simulink model "Pedal_Position_Sensor"  (R2021a)
settings: Solver=FixedStepAuto  StartTime=0.0  StopTime=10.0  RelTol=1e-3
libraries: simulink x3, pil_lib x2
settings Model: Creator=LenovoID3  LastModifiedBy=LenovoID3
settings OptimizationCC: DefaultParameterBehavior=Inlined  EnhancedBackFolding=on  PassReuseOutputArgsAs=Individual arguments  ZeroExternalMemoryAtStartup=off  ZeroInternalMemoryAtStartup=off  OptimizeBlockOrder=speed  DifferentSizesBufferReuse=on  OptimizationCustomize=off  EfficientTunableParamExpr=on
settings DebuggingCC: ParameterTunabilityLossMsg=error
settings SFSimCC: MATLABDynamicMemAlloc=off
settings RTWCC: SystemTargetFile=ert.tlc  TemplateMakefile=ert_default_tmf  CreateSILPILBlock=SIL
settings CodeAppCC: ForceParamTrailComments=on  IgnoreCustomStorageClasses=off  OperatorAnnotations=on  SimulinkDataObjDesc=on  SFDataObjDesc=on  InsertBlockDesc=on
settings ERTTargetCC: TargetLangStandard=C99 (ISO)  GenerateSampleERTMain=on  SupportContinuousTime=on  InlinedParameterPlacement=NonHierarchical  ERTCustomFileTemplate=example_file_process.tlc

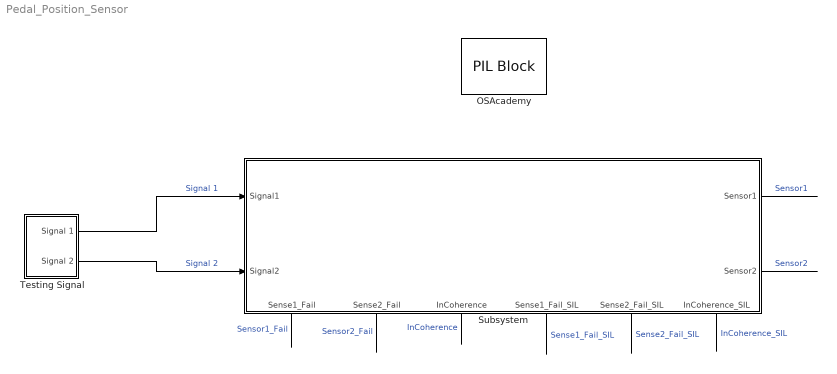
== system Pedal_Position_Sensor ==
  OSAcademy : pil_lib/PIL Block  SimulationMode=SIL  IsTopModelPIL=off  CodeDir=C:\Users\LenovoID3\Downloads\New folder\OSAcademy_ert_rtw  AnchorDir=C:\Users\LenovoID3\Downloads\New folder  ConfigName=Software-in-the-Loop (SIL)  XrelIsTopModelCode=on  XrelIsReusable=off  XrelDWorkNames={}  XrelDWorkTypes={}  XrelModelArgVals={}  XrelOrderedParamNames={}
      settings: SourceProductBaseCode=RT
  Subsystem : Subsystem
      settings: PortSchema="{\"entries\":[{\"content\":{\"sides\":[{\"content\":{\"connectorIds\":[\"In1\",\"In2\"]},\"type\":\"ConnectorPlacement.EquallySpacedRectSide\",\"uuid\":\"b8229edd-deda-40cf-ad5a-24b3db798bf7\"},{\"content\":{\"connectorIds\":[\"Out1\",\"Out2\"],\"side\":\"RIGHT\"},\"type\":\"ConnectorPlacement.EquallySpacedRectSide\",\"uuid\":\"8a2a6cfd-0422-46e1-aba6-13dd86feb93d\"},{\"content\":{\"connectorIds\":[],\"side\":\"TOP\"},\"type\":\"ConnectorPlacement.EquallySpacedRectSide\",\"uuid\":\"1ebd3a65-a67e-4261-83c1-f99d1798de09\"},{\"content\":{\"connectorIds\":[\"Out3\",\"Out4\",\"Out5\",\"Out6\",\"Out7\",\"Out8\"],\"side\":\"BOTTOM\"},\"type\":\"ConnectorPlacement.EquallySpacedRectSide\",\"uuid\":\"0ad3b253-8be6-4aef-90be-6048caeda625\"}]},\"type\":\"ConnectorPlacement.EquallySpacedConnector\",\"uuid\":\"11bd23d5-d2a7-463d-b28b-d598d29700f0\"}],\"packageUris\":[\"http://schema.mathworks.com/mf0/Connector/R2020b\"],\"version\":\"1.0\"}"
  Testing Signal : Subsystem
  wires:
  Subsystem/1(Sensor1) -> ?  "Sensor1"
  Subsystem/2(Sensor2) -> ?  "Sensor2"
  Subsystem/5(InCoherence) -> ?  "InCoherence"
  Subsystem/4(Sense2_Fail) -> ?  "Sensor2_Fail"
  Subsystem/3(Sense1_Fail) -> ?  "Sensor1_Fail"
  Subsystem/6(Sense1_Fail_SIL) -> ?  "Sense1_Fail_SIL"
  Subsystem/7(Sense2_Fail_SIL) -> ?  "Sense2_Fail_SIL"
  Subsystem/8(InCoherence_SIL) -> ?  "InCoherence_SIL"
  Testing Signal/1(Signal 1) -> Subsystem/1(Signal1)  "Signal 1"
  Testing Signal/2(Signal 2) -> Subsystem/2(Signal2)  "Signal 2"

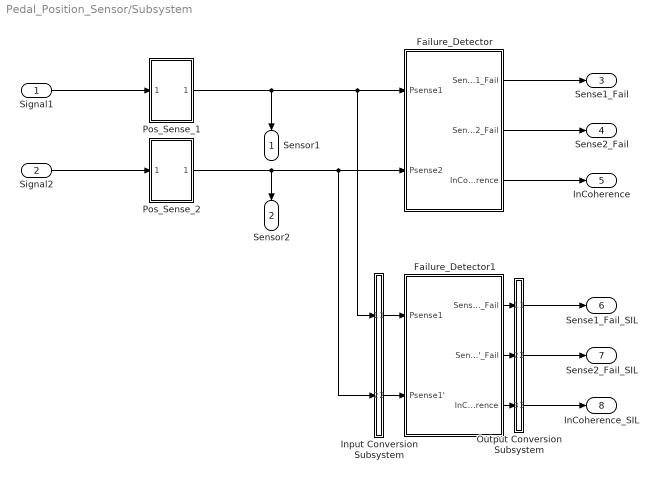
== system Pedal_Position_Sensor/Subsystem ==
  Signal1 : Inport
  Signal2 : Inport  Port=2
  Failure_Detector : Subsystem  TreatAsAtomicUnit=on
  Failure_Detector1 : Subsystem  Tag=__SL_testing_harness_stub_  DialogController=pil_create_dialog  LoadFcn=|
      | try
      |    if ~strcmp(rtw.pil.getPILVersion, '9.10 (R2021a)_15')
      |       set_param(gcb, 'DialogController', '');
      |       set_param(gcb, 'DialogControllerArgs', '');
      |    end
      | catch e
      |       set_param(gcb, 'DialogController', '');
      |       set_param(gcb, 'DialogControllerArgs', '');
      | end
      mask help: PIL:pil:XILBlockMaskDesc
      mask Display: disp('SIL');
  Input Conversion Subsystem : Subsystem  Tag=__SLT_ICS__  Description=|
      | Signal spec.
      | and routing
      settings: AttributesFormatString=%<Description>
  Output Conversion Subsystem : Subsystem  Tag=__SLT_OCS__  Description=|
      | Signal spec.
      | and routing
      settings: AttributesFormatString=%<Description>
  Pos_Sense_1 : Subsystem
  Pos_Sense_2 : Subsystem
  Sensor1 : Outport
  Sensor2 : Outport  Port=2
  Sense1_Fail : Outport  Port=3
  Sense2_Fail : Outport  Port=4
  InCoherence : Outport  Port=5
  Sense1_Fail_SIL : Outport  Port=6
  Sense2_Fail_SIL : Outport  Port=7
  InCoherence_SIL : Outport  Port=8
  wires:
  Failure_Detector/1(Sense1_Fail) -> Sense1_Fail/1
  Pos_Sense_2/1(Psense2) -> Sensor2/1, Input Conversion Subsystem/2(Inport_2), Failure_Detector/2(Psense2)
  Pos_Sense_1/1(Psense1) -> Sensor1/1, Input Conversion Subsystem/1(Inport_1), Failure_Detector/1(Psense1)
  Signal1/1 -> Pos_Sense_1/1(Input)
  Failure_Detector/3(InCoherence) -> InCoherence/1
  Failure_Detector/2(Sense2_Fail) -> Sense2_Fail/1
  Signal2/1 -> Pos_Sense_2/1(Input)
  Input Conversion Subsystem/2(Outport_2) -> Failure_Detector1/2(Psense1')
  Failure_Detector1/3(InCoherence) -> Output Conversion Subsystem/3(Inport_3)
  Output Conversion Subsystem/2(Outport_2) -> Sense2_Fail_SIL/1
  Failure_Detector1/1(Sense1_Fail) -> Output Conversion Subsystem/1(Inport_1)
  Input Conversion Subsystem/1(Outport_1) -> Failure_Detector1/1(Psense1)
  Output Conversion Subsystem/1(Outport_1) -> Sense1_Fail_SIL/1
  Output Conversion Subsystem/3(Outport_3) -> InCoherence_SIL/1
  Failure_Detector1/2(Sense1'_Fail) -> Output Conversion Subsystem/2(Inport_2)

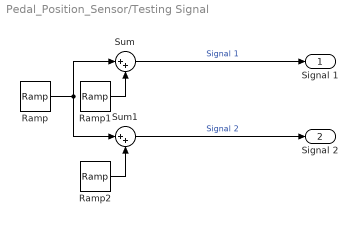
== system Pedal_Position_Sensor/Testing Signal ==
  Ramp : simulink/Sources/Ramp  slope=0.1  start=0  InitialOutput=0
  Ramp1 : simulink/Sources/Ramp  slope=0.2  start=5  InitialOutput=0
  Ramp2 : simulink/Sources/Ramp  slope=0.3  start=5  InitialOutput=0
  Sum : Sum  Inputs=|++
  Sum1 : Sum  Inputs=|++
  Signal 1 : Outport
  Signal 2 : Outport  Port=2
  wires:
  Ramp2/1 -> Sum1/2
  Ramp1/1 -> Sum/2
  Sum/1 -> Signal 1/1  "Signal 1"
  Sum1/1 -> Signal 2/1  "Signal 2"
  Ramp/1 -> Sum/1, Sum1/1

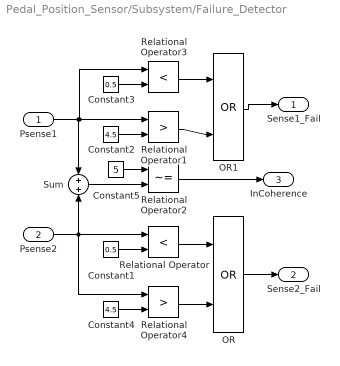
== system Pedal_Position_Sensor/Subsystem/Failure_Detector ==
  Psense1 : Inport
  Psense2 : Inport  Port=2
  Constant1 : Constant  Value=0.5
  Constant2 : Constant  Value=4.5
  Constant3 : Constant  Value=0.5
  Constant4 : Constant  Value=4.5
  Constant5 : Constant  Value=5
  OR : Logic  Operator=OR  AllPortsSameDT=off  OutDataTypeStr=boolean
  OR1 : Logic  Operator=OR  AllPortsSameDT=off  OutDataTypeStr=boolean
  Relational Operator : RelationalOperator  Operator=<  OutDataTypeStr=boolean  RndMeth=Simplest
  Relational Operator1 : RelationalOperator  Operator=>  OutDataTypeStr=boolean  RndMeth=Simplest
  Relational Operator2 : RelationalOperator  Operator=~=  OutDataTypeStr=boolean  RndMeth=Simplest
  Relational Operator3 : RelationalOperator  Operator=<  OutDataTypeStr=boolean  RndMeth=Simplest
  Relational Operator4 : RelationalOperator  Operator=>  OutDataTypeStr=boolean  RndMeth=Simplest
  Sum : Sum
  Sense1_Fail : Outport
  Sense2_Fail : Outport  Port=2
  InCoherence : Outport  Port=3
  wires:
  Constant1/1 -> Relational Operator/2
  Constant2/1 -> Relational Operator1/2
  Constant3/1 -> Relational Operator3/2
  Psense1/1 -> Relational Operator3/1, Relational Operator1/1, Sum/1
  Psense2/1 -> Relational Operator4/1, Sum/2, Relational Operator/1
  Constant4/1 -> Relational Operator4/2
  Relational Operator/1 -> OR/1
  Relational Operator4/1 -> OR/2
  Relational Operator1/1 -> OR1/2
  Relational Operator3/1 -> OR1/1
  OR1/1 -> Sense1_Fail/1
  OR/1 -> Sense2_Fail/1
  Relational Operator2/1 -> InCoherence/1
  Sum/1 -> Relational Operator2/2
  Constant5/1 -> Relational Operator2/1

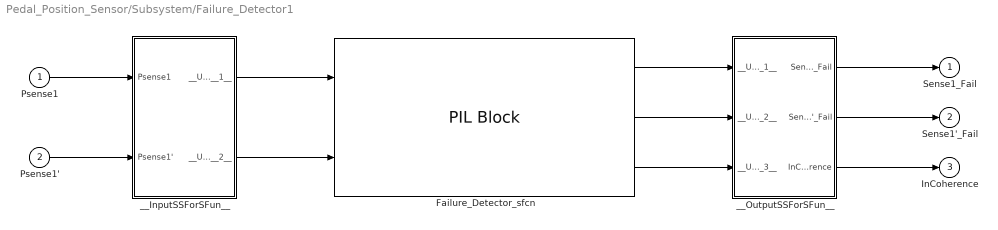
== system Pedal_Position_Sensor/Subsystem/Failure_Detector1 ==
  Psense1 : Inport
  Psense1' : Inport  Port=2
  Failure_Detector_sfcn : pil_lib/PIL Block  SimulationMode=SIL  IsTopModelPIL=off  CodeDir=C:\Users\LenovoID3\Downloads\New folder\Failure_Detector_ert_rtw  AnchorDir=C:\Users\LenovoID3\Downloads\New folder  ConfigName=Software-in-the-Loop (SIL)  XrelIsTopModelCode=on  XrelIsReusable=off  XrelDWorkNames={}  XrelDWorkTypes={}  XrelModelArgVals={}  XrelOrderedParamNames={}
      settings: SourceProductBaseCode=RT
  __InputSSForSFun__ : Subsystem
  __OutputSSForSFun__ : Subsystem
  Sense1_Fail : Outport
  Sense1'_Fail : Outport  Port=2
  InCoherence : Outport  Port=3
  wires:
  __OutputSSForSFun__/3(InCoherence) -> InCoherence/1
  __OutputSSForSFun__/2(Sense1'_Fail) -> Sense1'_Fail/1
  __OutputSSForSFun__/1(Sense1_Fail) -> Sense1_Fail/1
  Failure_Detector_sfcn/3 -> __OutputSSForSFun__/3(__UniqueInportName__3__)
  Failure_Detector_sfcn/2 -> __OutputSSForSFun__/2(__UniqueInportName__2__)
  Failure_Detector_sfcn/1 -> __OutputSSForSFun__/1(__UniqueInportName__1__)
  __InputSSForSFun__/2(__UniqueOutportName__2__) -> Failure_Detector_sfcn/2
  __InputSSForSFun__/1(__UniqueOutportName__1__) -> Failure_Detector_sfcn/1
  Psense1'/1 -> __InputSSForSFun__/2(Psense1')
  Psense1/1 -> __InputSSForSFun__/1(Psense1)

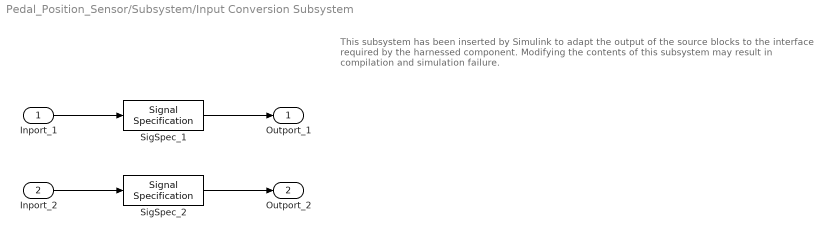
== system Pedal_Position_Sensor/Subsystem/Input Conversion Subsystem ==
  note: This subsystem has been inserted by Simulink to adapt the output of the source blocks to the interface required by the harnessed component.
      |  Modifying the contents of this subsystem may result in compilation and simulation failure.
  Inport_1 : Inport
  Inport_2 : Inport  Port=2
  SigSpec_1 : SignalSpecification  OutDataTypeStr=double  Dimensions=[1]  SampleTime=[0, 0]
  SigSpec_2 : SignalSpecification  OutDataTypeStr=double  Dimensions=[1]  SampleTime=[0, 0]
  Outport_1 : Outport
  Outport_2 : Outport  Port=2
  wires:
  SigSpec_1/1 -> Outport_1/1
  Inport_1/1 -> SigSpec_1/1
  SigSpec_2/1 -> Outport_2/1
  Inport_2/1 -> SigSpec_2/1

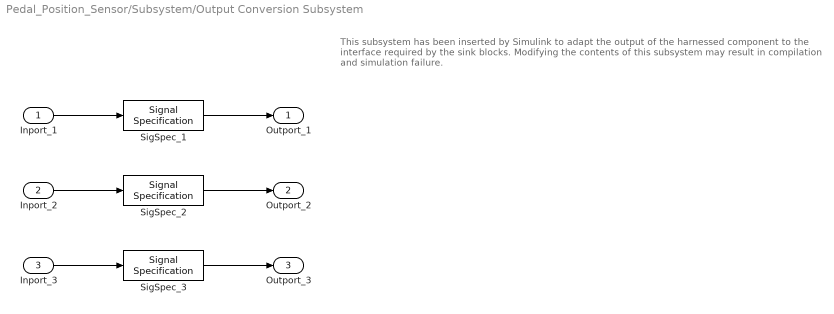
== system Pedal_Position_Sensor/Subsystem/Output Conversion Subsystem ==
  note: This subsystem has been inserted by Simulink to adapt the output of the harnessed component to the interface required by the sink blocks.
      |  Modifying the contents of this subsystem may result in compilation and simulation failure.
  Inport_1 : Inport
  Inport_2 : Inport  Port=2
  Inport_3 : Inport  Port=3
  SigSpec_1 : SignalSpecification  OutDataTypeStr=boolean  Dimensions=[1]
  SigSpec_2 : SignalSpecification  OutDataTypeStr=boolean  Dimensions=[1]
  SigSpec_3 : SignalSpecification  OutDataTypeStr=boolean  Dimensions=[1]
  Outport_1 : Outport
  Outport_2 : Outport  Port=2
  Outport_3 : Outport  Port=3
  wires:
  Inport_1/1 -> SigSpec_1/1
  SigSpec_1/1 -> Outport_1/1
  Inport_2/1 -> SigSpec_2/1
  SigSpec_2/1 -> Outport_2/1
  Inport_3/1 -> SigSpec_3/1
  SigSpec_3/1 -> Outport_3/1

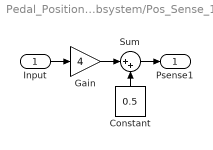
== system Pedal_Position_Sensor/Subsystem/Pos_Sense_1 ==
  Input : Inport
  Constant : Constant  Value=0.5
  Gain : Gain  Gain=4
  Sum : Sum  Inputs=|++
  Psense1 : Outport
  wires:
  Constant/1 -> Sum/2
  Gain/1 -> Sum/1
  Sum/1 -> Psense1/1
  Input/1 -> Gain/1

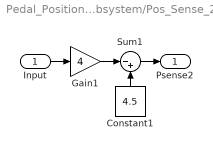
== system Pedal_Position_Sensor/Subsystem/Pos_Sense_2 ==
  Input : Inport
  Constant1 : Constant  Value=4.5
  Gain1 : Gain  Gain=4
  Sum1 : Sum  Inputs=|-+
  Psense2 : Outport
  wires:
  Gain1/1 -> Sum1/1
  Sum1/1 -> Psense2/1
  Constant1/1 -> Sum1/2
  Input/1 -> Gain1/1

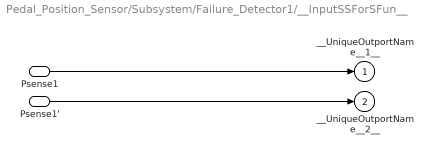
== system Pedal_Position_Sensor/Subsystem/Failure_Detector1/__InputSSForSFun__ ==
  Psense1 : Inport
  Psense1' : Inport  Port=2
  __UniqueOutportName__1__ : Outport
  __UniqueOutportName__2__ : Outport  Port=2
  wires:
  Psense1'/1 -> __UniqueOutportName__2__/1
  Psense1/1 -> __UniqueOutportName__1__/1

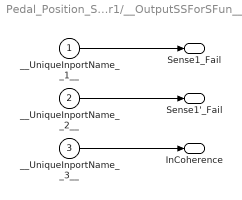
== system Pedal_Position_Sensor/Subsystem/Failure_Detector1/__OutputSSForSFun__ ==
  __UniqueInportName__1__ : Inport
  __UniqueInportName__2__ : Inport  Port=2
  __UniqueInportName__3__ : Inport  Port=3
  Sense1_Fail : Outport
  Sense1'_Fail : Outport  Port=2
  InCoherence : Outport  Port=3
  wires:
  __UniqueInportName__3__/1 -> InCoherence/1
  __UniqueInportName__2__/1 -> Sense1'_Fail/1
  __UniqueInportName__1__/1 -> Sense1_Fail/1
